simulink model "exp5_pwdModulator"  (R2023b)
settings: Solver=VariableStepAuto  StartTime=0.0  StopTime=0.01  RelTol=1e-3
settings Model: Creator=ketaki mahajan  LastModifiedBy=ketaki mahajan

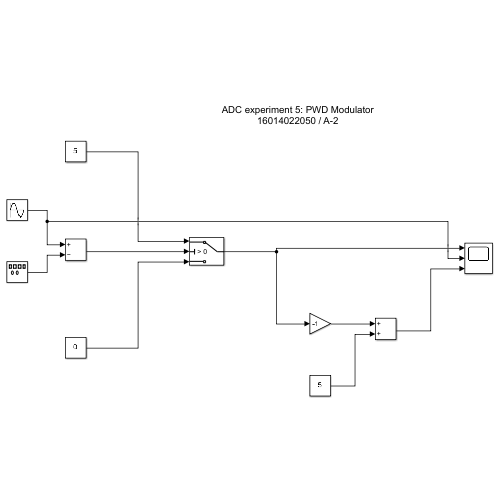
[thumbnail: Simulink's stored preview of the top-level diagram]
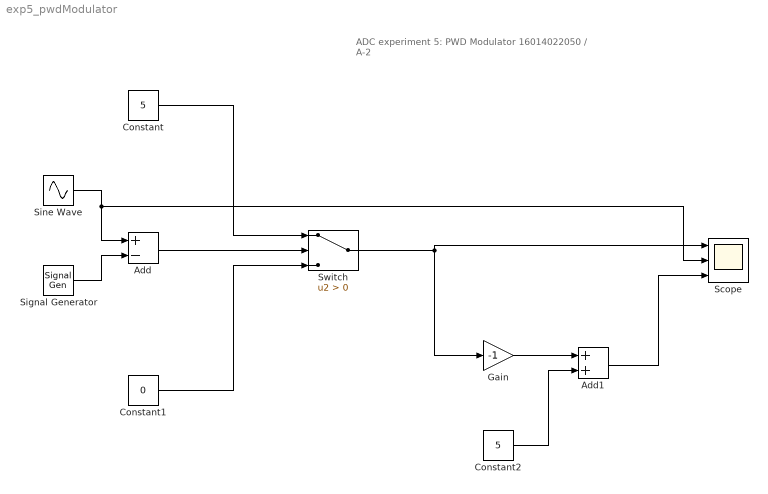
== system exp5_pwdModulator ==
  note: ADC experiment 5: PWD Modulator
      | 16014022050 / A-2
  Add : Sum  Inputs=+-
  Add1 : Sum
  Constant : Constant  Value=5
  Constant1 : Constant  Value=0
  Constant2 : Constant  Value=5
  Gain : Gain  Gain=-1
  Scope : Scope  NumInputPorts=3
  Signal Generator : SignalGenerator  WaveForm=sawtooth  Amplitude=5  Frequency=10000
  Sine Wave : Sin  Amplitude=5  Frequency=6283.183  SampleTime=0
  Switch : Switch  Criteria=u2 > Threshold  SaturateOnIntegerOverflow=off  InputSameDT=off
  wires:
  Sine Wave/1 -> Scope/2, Add/1
  Signal Generator/1 -> Add/2
  Add/1 -> Switch/2
  Constant/1 -> Switch/1
  Constant1/1 -> Switch/3
  Switch/1 -> Gain/1, Scope/1
  Gain/1 -> Add1/1
  Constant2/1 -> Add1/2
  Add1/1 -> Scope/3
